simulink model "AtomicTestDiscrete_inest"  (R2017a)
settings: Solver=FixedStepDiscrete  StartTime=0.0  StopTime=.2  FixedStep=1e-6  RelTol=1e-3
undefined symbols (not defined in the file or in its folder): DiscIntNeverNeededParam
settings Model: Creator=erich  LastModifiedBy=erich

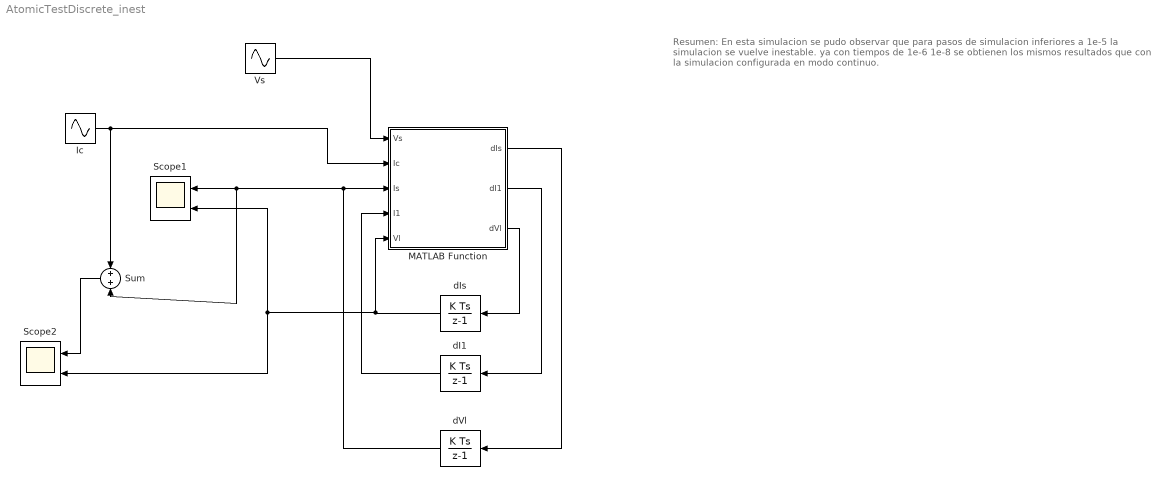
== system AtomicTestDiscrete_inest ==
  note: Resumen:
      | En esta simulacion se pudo observar que para pasos de simulacion
      | inferiores a 1e-5 la simulacion se vuelve inestable. ya con tiempos de
      | 1e-6 1e-8 se obtienen los mismos resultados que con la simulacion
      | configurada en modo continuo.
  Ic : Sin  Amplitude=50  Frequency=2*pi*60  Phase=-2*pi/5  SampleTime=0
  MATLAB Function : MATLAB Function  TreatAsAtomicUnit=on
  Scope1 : Scope  NumInputPorts=2
  Scope2 : Scope  NumInputPorts=2
  Sum : Sum  Inputs=+|+
  Vs : Sin  Amplitude=170  Frequency=2*pi*60  SampleTime=0
  dI1 : DiscreteIntegrator  gainval=1  InitialConditionSetting=State (most efficient)  SampleTime=-1  ICPrevOutput=DiscIntNeverNeededParam  ICPrevScaledInput=DiscIntNeverNeededParam
  dIs : DiscreteIntegrator  gainval=1  InitialConditionSetting=State (most efficient)  SampleTime=-1  ICPrevOutput=DiscIntNeverNeededParam  ICPrevScaledInput=DiscIntNeverNeededParam
  dVl : DiscreteIntegrator  gainval=1  InitialConditionSetting=State (most efficient)  SampleTime=-1  ICPrevOutput=DiscIntNeverNeededParam  ICPrevScaledInput=DiscIntNeverNeededParam
  wires:
  Sum/1 -> Scope2/1
  dVl/1 -> Sum/2, Scope1/1, MATLAB Function/3(Is)
  MATLAB Function/2(dI1) -> dI1/1
  dI1/1 -> MATLAB Function/4(I1)
  Ic/1 -> Sum/1, MATLAB Function/2(Ic)
  MATLAB Function/3(dVl) -> dIs/1
  Vs/1 -> MATLAB Function/1(Vs)
  MATLAB Function/1(dIs) -> dVl/1
  dIs/1 -> Scope1/2, Scope2/2, MATLAB Function/5(Vl)

== matlab function AtomicTestDiscrete_inest/MATLAB Function ==
  data: Vs input; dIs output; Ic input; Is input; I1 input; Vl input; dI1 output; dVl output
function [dIs, dI1, dVl] = fcn(Vs, Ic, Is, I1, Vl)

% parametros
rs = 1e-3; % parte resistiva impedancia de linea
Ls = 1e-6; % parte inductiva impedancia de linea

% valores de los componentes de la carga.
Cl = 2000e-6;
Ll = 5.2;
rl = 10; 
Rl = 10;

dIs = ((Vs-Vl)-Is*rs)/Ls;

dI1 = (Vl - I1*rl)/Ll;

dVl = ( (Ic+Is) -I1 -(Vl/Rl) )/Cl;
